simulink model "hdv_hydroelectropowertrain_model"  (R2023b)
settings: Solver=ode1be  StartTime=0.0  StopTime=simulation_length  FixedStep=tsample  MaxStep=tsample
values from neighbouring files (symbols this model uses):
  alpha = 35    [init_model.m]
  Apump = [0 1; 0 0]    [init_model.m]
  available_torque = torque_base+torque_friction_base    [init_model.m]
  Bpump = [0 1]'    [init_model.m]
  btheta_shaft = 2e2    (= 200)    [init_model.m]
  C1 = 10    [init_model.m]
  consumption = [consumption_1, consumption_2, consumption_3, consumption_4,          consumption_5, consumption_6, consumption_7, consumption_8,          consumption_9, consumption_10, consumption_11, consumption_12,          consumption_13, consumption_14, consumption_15, consumption_16          ]    [ic_engine_data.m]
  Cpump = [k 0]    [init_model.m]
  dp_lim = 400    [init_model.m]
  E0 = 3.685    [init_model.m]
  E1 = 0.2156    [init_model.m]
  E2 = 0    [init_model.m]
  E3 = 0    [init_model.m]
  E_1 = -1.031    [init_model.m]
  Elog = -0.05    [init_model.m]
  eta_v_m = 0.98    [init_model.m]
  eta_v_p = 0.97    [init_model.m]
  ki_dp_comp = 1/dp_lim    (= 0.0025)    [init_model.m]
  ki_te_comp = 2/te_lim    [init_model.m]
  kp_ctrl_m = 1    [init_model.m]
  kp_dp_comp = 0.5/dp_lim    (= 0.00125)    [init_model.m]
  kp_te_comp = 1/te_lim    [init_model.m]
  Kpump = acker(Apump,Bpump,poles)    [init_model.m]
  load_blade_enable = 0    [init_model.m]
  Lpump = acker(Apump',Cpump',pole_so)'    [init_model.m]
  M = 125    [init_model.m]
  Ncell = 185    [init_model.m]
  Npump = -1/(Cpump*inv(Apump-Bpump*Kpump)*Bpump)    [init_model.m]
  omega_e_rpm_ref = 1700    [init_model.m]
  omega_l_max_rpm = omega_l_max/(2*pi)*60    (= 50.3075969543)    [init_model.m]
  q1Kalman = tsample^2*1e-2    (= 1e-08)    [init_model.m]
  q2Kalman = tsample^1*1e-1    (= 0.0001)    [init_model.m]
  q3Kalman = 0    [init_model.m]
  Qhr = 400    [init_model.m]
  R0 = 0.015    [init_model.m]
  R1 = 0.015    [init_model.m]
  R_tg = 1.16/2    (= 0.58)    [init_model.m]
  rKalman = 1    [init_model.m]
  rpm_base = [620 700 800 900 1000 1100 1200 1300 1400 1500 1600 1700 1800      1900 2000 2100]    [ic_engine_data.m]
  rpm_consumption = rpm_base    [ic_engine_data.m]
  simulation_length = 245    [init_model.m]
  tau_load = 75e3    (= 75000)    [init_model.m]
  tau_load_max = 1600*41.4    (= 66240)    [init_model.m]
  Tc = tsample    (= 0.001)    [init_model.m]
  torque_base = [max(torque_16_data) max(torque_15_data) max(torque_14_data)      max(torque_13_data) max(torque_12_data) max(torque_11_data)      max(torque_10_data) max(torque_9_data) max(torque_8_data)      max(torque_7_data) max(torque_6_data) max(torque_5_data)      max(torque_4_data) max(torque_3_data) max(torque_2_data)      max(torque_1_data)]    [ic_engine_data.m]
  torque_consumption = torque_reference    [ic_engine_data.m]
  torque_friction_base = -(rpm_base./60*2*pi)*0.25-(rpm_base./60*2*pi).^2*5.2e-4    [ic_engine_data.m]
  tsample = 1e-3    (= 0.001)    [init_model.m]
  v_track1_ref = 8    [init_model.m]
  v_track2_ref = 8    [init_model.m]
  valve_mmorifice_max = 2.75    [init_model.m]
  xv_m_max = 1.2    [init_model.m]
undefined symbols (not defined in the file or in its folder): magnitude
libraries: fl_lib x381, nesl_utility x162, linear_swashplate_ctrl_lib x8, flexshaft_lib x5, bichamber_piston_lib x5, variable_displacement_motor_lib x4, variable_displacement_pump_lib x4, fixed_displacement_pump_lib x4, relief_valve_lib x4, inverse_shuttle_valve_lib x4, hydrostatic_threeway_valve_bichamber_piston_lib x4, hydrostatic_fourway_valve_bichamber_piston_lib x4
(part 4 of 9)

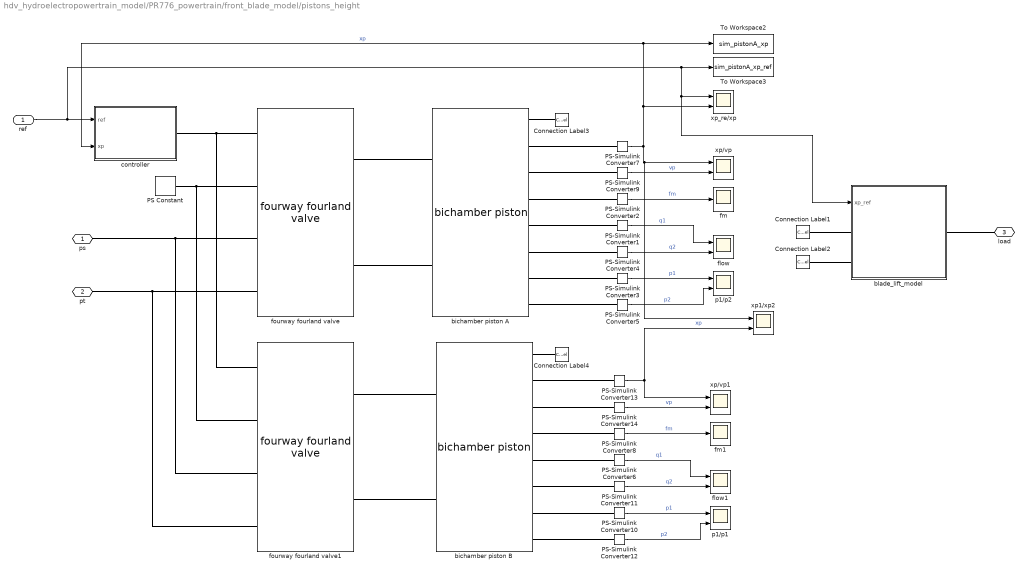
== system hdv_hydroelectropowertrain_model/PR776_powertrain/front_blade_model/pistons_height ==
  ref : Inport
  Connection Label1 : ConnectionLabel  Label=A
  Connection Label2 : ConnectionLabel  Label=B
  Connection Label3 : ConnectionLabel  Label=A
  Connection Label4 : ConnectionLabel  Label=B
  PS Constant : fl_lib/Physical Signals/Sources/PS Constant  constant=0 mm
  PS-Simulink Converter{1..14} (14 alike) : nesl_utility/PS-Simulink Converter  PhysicalDomain=network_engine_domain  SubClassName=ps_output  LeftPortType=input  RightPortType=output  PseudoPeriodic=off  Frequencies=[]  VectorFormat=1-D array  Unit=inherit  AffineConversion=off
  To Workspace2 : ToWorkspace  VariableName=sim_pistonA_xp  SampleTime=Tc
      settings: MaxDataPoints=Nc
  To Workspace3 : ToWorkspace  VariableName=sim_pistonA_xp_ref  SampleTime=Tc
      settings: MaxDataPoints=Nc
  bichamber piston A : bichamber_piston_lib/bichamber piston  A1=8e-3 m^2  A2=8e-3 m^2  Lp=1 m  mp=35 kg  kp=0 N/m  bp=1e3 N/(m/s)  V0=12 l  q1_specify=off  q1_priority=None  q1=0 m^3/s  q1_nominal_specify=off  q1_nominal_unit=m^3/s  q1_nominal_value=1  q2_specify=off  q2_priority=None  q2=0 m^3/s  q2_nominal_specify=off  q2_nominal_unit=m^3/s  q2_nominal_value=1  p1_specify=off  p1_priority=High  p1=0 bar  p1_nominal_specify=off  p1_nominal_unit=bar  p1_nominal_value=1  p2_specify=off  p2_priority=High  p2=125 bar  p2_nominal_specify=off  p2_nominal_unit=bar  p2_nominal_value=1  fp_specify=off  fp_priority=None  fp=0 N  fp_nominal_specify=off  fp_nominal_unit=N  fp_nominal_value=1  vp_specify=off  vp_priority=None  vp=0 m/s  vp_nominal_specify=off  vp_nominal_unit=m/s  vp_nominal_value=1  xp_specify=off  xp_priority=High  xp=0 m  xp_nominal_specify=off  xp_nominal_unit=m  xp_nominal_value=1
      settings: InternalSimscapePortConfiguration="{\"Bottom\":[],\"Left\":[{\"id\":\"H1\",\"label\":\"H1\",\"type\":\"foundation.hydraulic.hydraulic\"},{\"id\":\"H2\",\"label\":\"H2\",\"type\":\"foundation.hydraulic.hydraulic\"}],\"Right\":[{\"id\":\"P\",\"label\":\"P\",\"type\":\"foundation.mechanical.translational.translational\"},{\"id\":\"xp_out\",\"label\":\"xp\",\"type\":\"output\"},{\"id\":\"vp_out\",\"label\":\"vp\",\"type\":\"output\"},{\"id\":\"mforce\",\"label\":\"fm\",\"type\":\"output\"},{\"id\":\"q1_out\",\"label\":\"q1\",\"type\":\"output\"},{\"id\":\"q2_out\",\"label\":\"q2\",\"type\":\"output\"},{\"id\":\"p1_out\",\"label\":\"p1\",\"type\":\"output\"},{\"id\":\"p2_out\",\"label\":\"p2\",\"type\":\"output\"}],\"Top\":[]}"
  bichamber piston B : bichamber_piston_lib/bichamber piston  A1=8e-3 m^2  A2=8e-3 m^2  Lp=1 m  mp=35 kg  kp=0 N/m  bp=1e3 N/(m/s)  V0=12 l  q1_specify=off  q1_priority=None  q1=0 m^3/s  q1_nominal_specify=off  q1_nominal_unit=m^3/s  q1_nominal_value=1  q2_specify=off  q2_priority=None  q2=0 m^3/s  q2_nominal_specify=off  q2_nominal_unit=m^3/s  q2_nominal_value=1  p1_specify=off  p1_priority=High  p1=0 bar  p1_nominal_specify=off  p1_nominal_unit=bar  p1_nominal_value=1  p2_specify=off  p2_priority=High  p2=125 bar  p2_nominal_specify=off  p2_nominal_unit=bar  p2_nominal_value=1  fp_specify=off  fp_priority=None  fp=0 N  fp_nominal_specify=off  fp_nominal_unit=N  fp_nominal_value=1  vp_specify=off  vp_priority=None  vp=0 m/s  vp_nominal_specify=off  vp_nominal_unit=m/s  vp_nominal_value=1  xp_specify=off  xp_priority=High  xp=0 m  xp_nominal_specify=off  xp_nominal_unit=m  xp_nominal_value=1
      settings: InternalSimscapePortConfiguration="{\"Bottom\":[],\"Left\":[{\"id\":\"H1\",\"label\":\"H1\",\"type\":\"foundation.hydraulic.hydraulic\"},{\"id\":\"H2\",\"label\":\"H2\",\"type\":\"foundation.hydraulic.hydraulic\"}],\"Right\":[{\"id\":\"P\",\"label\":\"P\",\"type\":\"foundation.mechanical.translational.translational\"},{\"id\":\"xp_out\",\"label\":\"xp\",\"type\":\"output\"},{\"id\":\"vp_out\",\"label\":\"vp\",\"type\":\"output\"},{\"id\":\"mforce\",\"label\":\"fm\",\"type\":\"output\"},{\"id\":\"q1_out\",\"label\":\"q1\",\"type\":\"output\"},{\"id\":\"q2_out\",\"label\":\"q2\",\"type\":\"output\"},{\"id\":\"p1_out\",\"label\":\"p1\",\"type\":\"output\"},{\"id\":\"p2_out\",\"label\":\"p2\",\"type\":\"output\"}],\"Top\":[]}"
  blade_lift_model : Subsystem
  controller : Subsystem
  flow : Scope  NumInputPorts=2
  flow1 : Scope  NumInputPorts=2
  fm : Scope
  fm1 : Scope
  fourway fourland valve : fourway_fourland_valve_lib/fourway fourland valve  xv_max=valve_mmorifice_max mm  ps_specify=off  ps_priority=None  ps=0 bar  ps_nominal_specify=off  ps_nominal_unit=bar  ps_nominal_value=1  pt_specify=off  pt_priority=None  pt=0 bar  pt_nominal_specify=off  pt_nominal_unit=bar  pt_nominal_value=1  q1_specify=off  q1_priority=None  q1=0 m^3/s  q1_nominal_specify=off  q1_nominal_unit=m^3/s  q1_nominal_value=1  q2_specify=off  q2_priority=None  q2=0 m^3/s  q2_nominal_specify=off  q2_nominal_unit=m^3/s  q2_nominal_value=1  q3_specify=off  q3_priority=None  q3=0 m^3/s  q3_nominal_specify=off  q3_nominal_unit=m^3/s  q3_nominal_value=1  q4_specify=off  q4_priority=None  q4=0 m^3/s  q4_nominal_specify=off  q4_nominal_unit=m^3/s  q4_nominal_value=1  q5_specify=off  q5_priority=None  q5=0 m^3/s  q5_nominal_specify=off  q5_nominal_unit=m^3/s  q5_nominal_value=1  q6_specify=off  q6_priority=None  q6=0 m^3/s  q6_nominal_specify=off  q6_nominal_unit=m^3/s  q6_nominal_value=1  qs_specify=off  qs_priority=None  qs=0 m^3/s  qs_nominal_specify=off  qs_nominal_unit=m^3/s  qs_nominal_value=1  qt_specify=off  qt_priority=None  qt=0 m^3/s  qt_nominal_specify=off  qt_nominal_unit=m^3/s  qt_nominal_value=1  p1_specify=off  p1_priority=High  p1=125 bar  p1_nominal_specify=off  p1_nominal_unit=bar  p1_nominal_value=1  p2_specify=off  p2_priority=High  p2=125 bar  p2_nominal_specify=off  p2_nominal_unit=bar  p2_nominal_value=1
      settings: InternalSimscapePortConfiguration="{\"Bottom\":[],\"Left\":[{\"id\":\"xv\",\"label\":\"xv\",\"type\":\"input\"},{\"id\":\"x0\",\"label\":\"x0\",\"type\":\"input\"},{\"id\":\"S\",\"label\":\"S\",\"type\":\"foundation.hydraulic.hydraulic\"},{\"id\":\"T\",\"label\":\"T\",\"type\":\"foundation.hydraulic.hydraulic\"}],\"Right\":[{\"id\":\"H1\",\"label\":\"H1\",\"type\":\"foundation.hydraulic.hydraulic\"},{\"id\":\"H2\",\"label\":\"H2\",\"type\":\"foundation.hydraulic.hydraulic\"}],\"Top\":[]}"
  fourway fourland valve1 : fourway_fourland_valve_lib/fourway fourland valve  xv_max=valve_mmorifice_max mm  ps_specify=off  ps_priority=None  ps=0 bar  ps_nominal_specify=off  ps_nominal_unit=bar  ps_nominal_value=1  pt_specify=off  pt_priority=None  pt=0 bar  pt_nominal_specify=off  pt_nominal_unit=bar  pt_nominal_value=1  q1_specify=off  q1_priority=None  q1=0 m^3/s  q1_nominal_specify=off  q1_nominal_unit=m^3/s  q1_nominal_value=1  q2_specify=off  q2_priority=None  q2=0 m^3/s  q2_nominal_specify=off  q2_nominal_unit=m^3/s  q2_nominal_value=1  q3_specify=off  q3_priority=None  q3=0 m^3/s  q3_nominal_specify=off  q3_nominal_unit=m^3/s  q3_nominal_value=1  q4_specify=off  q4_priority=None  q4=0 m^3/s  q4_nominal_specify=off  q4_nominal_unit=m^3/s  q4_nominal_value=1  q5_specify=off  q5_priority=None  q5=0 m^3/s  q5_nominal_specify=off  q5_nominal_unit=m^3/s  q5_nominal_value=1  q6_specify=off  q6_priority=None  q6=0 m^3/s  q6_nominal_specify=off  q6_nominal_unit=m^3/s  q6_nominal_value=1  qs_specify=off  qs_priority=None  qs=0 m^3/s  qs_nominal_specify=off  qs_nominal_unit=m^3/s  qs_nominal_value=1  qt_specify=off  qt_priority=None  qt=0 m^3/s  qt_nominal_specify=off  qt_nominal_unit=m^3/s  qt_nominal_value=1  p1_specify=off  p1_priority=High  p1=125 bar  p1_nominal_specify=off  p1_nominal_unit=bar  p1_nominal_value=1  p2_specify=off  p2_priority=High  p2=125 bar  p2_nominal_specify=off  p2_nominal_unit=bar  p2_nominal_value=1
      settings: InternalSimscapePortConfiguration="{\"Bottom\":[],\"Left\":[{\"id\":\"xv\",\"label\":\"xv\",\"type\":\"input\"},{\"id\":\"x0\",\"label\":\"x0\",\"type\":\"input\"},{\"id\":\"S\",\"label\":\"S\",\"type\":\"foundation.hydraulic.hydraulic\"},{\"id\":\"T\",\"label\":\"T\",\"type\":\"foundation.hydraulic.hydraulic\"}],\"Right\":[{\"id\":\"H1\",\"label\":\"H1\",\"type\":\"foundation.hydraulic.hydraulic\"},{\"id\":\"H2\",\"label\":\"H2\",\"type\":\"foundation.hydraulic.hydraulic\"}],\"Top\":[]}"
  p1/p1 : Scope  NumInputPorts=2
  p1/p2 : Scope  NumInputPorts=2
  xp/vp : Scope  NumInputPorts=2
  xp/vp1 : Scope  NumInputPorts=2
  xp1/xp2 : Scope  NumInputPorts=2
  xp_re/xp : Scope  NumInputPorts=2
  ps : PMIOPort  Side=Left
  pt : PMIOPort  Port=2  Side=Left
  load : PMIOPort  Port=3  Side=Right
  wires:
  PS-Simulink Converter3/1 -> p1/p2/1  "p1"
  PS-Simulink Converter7/1 -> controller/2(xp), To Workspace2/1, xp_re/xp/2, xp1/xp2/1, xp/vp/1  "xp"
  PS-Simulink Converter4/1 -> flow/2  "q2"
  PS-Simulink Converter9/1 -> xp/vp/2  "vp"
  PS-Simulink Converter5/1 -> p1/p2/2  "p2"
  PS-Simulink Converter1/1 -> flow/1  "q1"
  PS-Simulink Converter2/1 -> fm/1  "fm"
  PS-Simulink Converter8/1 -> fm1/1  "fm"
  PS-Simulink Converter6/1 -> flow1/1  "q1"
  PS-Simulink Converter12/1 -> p1/p1/2  "p2"
  PS-Simulink Converter14/1 -> xp/vp1/2  "vp"
  PS-Simulink Converter11/1 -> flow1/2  "q2"
  PS-Simulink Converter13/1 -> xp1/xp2/2, xp/vp1/1  "xp"
  PS-Simulink Converter10/1 -> p1/p1/1  "p1"
  ref/1 -> blade_lift_model/1(xp_ref), xp_re/xp/1, To Workspace3/1, controller/1(ref)
  connections:
  bichamber piston A/RConn2 -- PS-Simulink Converter7/LConn1
  bichamber piston A/RConn3 -- PS-Simulink Converter9/LConn1
  bichamber piston A/RConn4 -- PS-Simulink Converter2/LConn1
  bichamber piston A/RConn5 -- PS-Simulink Converter1/LConn1
  bichamber piston A/RConn6 -- PS-Simulink Converter4/LConn1
  bichamber piston A/RConn7 -- PS-Simulink Converter3/LConn1
  bichamber piston A/RConn8 -- PS-Simulink Converter5/LConn1
  bichamber piston A/LConn1 -- fourway fourland valve/RConn1
  bichamber piston A/LConn2 -- fourway fourland valve/RConn2
  ps/RConn1 -- fourway fourland valve1/LConn3 -- fourway fourland valve/LConn3
  pt/RConn1 -- fourway fourland valve1/LConn4 -- fourway fourland valve/LConn4
  controller/RConn1 -- fourway fourland valve1/LConn1 -- fourway fourland valve/LConn1
  PS Constant/RConn1 -- fourway fourland valve/LConn2 -- fourway fourland valve1/LConn2
  bichamber piston B/RConn7 -- PS-Simulink Converter10/LConn1
  bichamber piston B/RConn5 -- PS-Simulink Converter6/LConn1
  bichamber piston B/RConn8 -- PS-Simulink Converter12/LConn1
  bichamber piston B/RConn4 -- PS-Simulink Converter8/LConn1
  bichamber piston B/RConn2 -- PS-Simulink Converter13/LConn1
  bichamber piston B/RConn3 -- PS-Simulink Converter14/LConn1
  bichamber piston B/RConn6 -- PS-Simulink Converter11/LConn1
  fourway fourland valve1/RConn1 -- bichamber piston B/LConn1
  fourway fourland valve1/RConn2 -- bichamber piston B/LConn2
  Connection Label3/LConn1 -- bichamber piston A/RConn1
  Connection Label4/LConn1 -- bichamber piston B/RConn1
  Connection Label1/LConn1 -- blade_lift_model/LConn1
  load/RConn1 -- blade_lift_model/RConn1
  Connection Label2/LConn1 -- blade_lift_model/LConn2

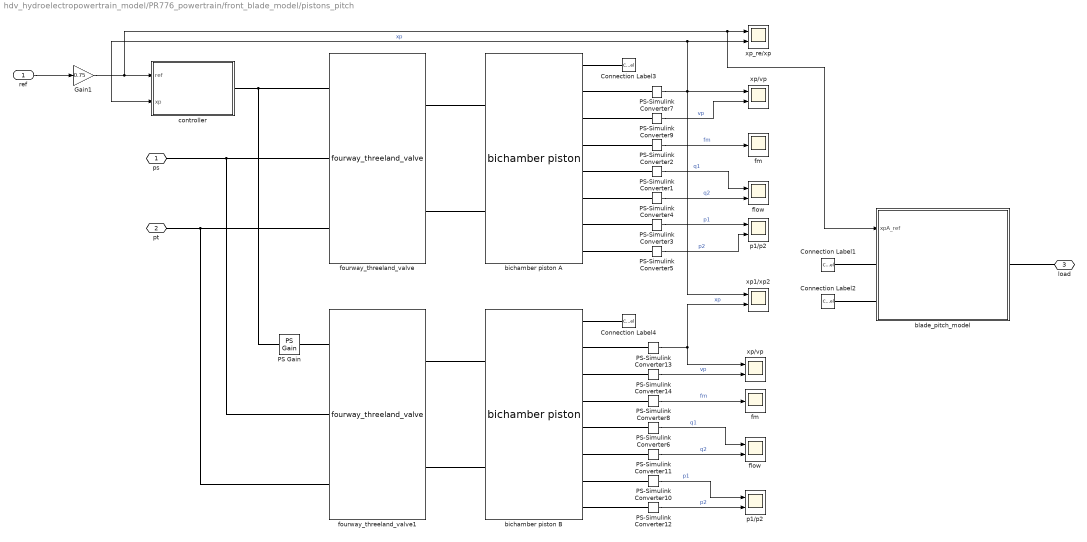
== system hdv_hydroelectropowertrain_model/PR776_powertrain/front_blade_model/pistons_pitch ==
  ref : Inport
  Connection Label1 : ConnectionLabel  Label=A
  Connection Label2 : ConnectionLabel  Label=B
  Connection Label3 : ConnectionLabel  Label=A
  Connection Label4 : ConnectionLabel  Label=B
  Gain1 : Gain  Gain=0.75
  PS Gain : fl_lib/Physical Signals/Functions/PS Gain  gain=-1
  PS-Simulink Converter{1..14} (14 alike) : nesl_utility/PS-Simulink Converter  PhysicalDomain=network_engine_domain  SubClassName=ps_output  LeftPortType=input  RightPortType=output  PseudoPeriodic=off  Frequencies=[]  VectorFormat=1-D array  Unit=inherit  AffineConversion=off
  bichamber piston A : bichamber_piston_lib/bichamber piston  A1=8e-3 m^2  A2=8e-3 m^2  Lp=1.1 m  mp=35 kg  kp=0 N/m  bp=1e3 N/(m/s)  V0=12 l  q1_specify=off  q1_priority=None  q1=0 m^3/s  q1_nominal_specify=off  q1_nominal_unit=m^3/s  q1_nominal_value=1  q2_specify=off  q2_priority=None  q2=0 m^3/s  q2_nominal_specify=off  q2_nominal_unit=m^3/s  q2_nominal_value=1  p1_specify=off  p1_priority=High  p1=0 bar  p1_nominal_specify=off  p1_nominal_unit=bar  p1_nominal_value=1  p2_specify=off  p2_priority=High  p2=0 bar  p2_nominal_specify=off  p2_nominal_unit=bar  p2_nominal_value=1  fp_specify=off  fp_priority=None  fp=0 N  fp_nominal_specify=off  fp_nominal_unit=N  fp_nominal_value=1  vp_specify=off  vp_priority=None  vp=0 m/s  vp_nominal_specify=off  vp_nominal_unit=m/s  vp_nominal_value=1  xp_specify=off  xp_priority=High  xp=0 m  xp_nominal_specify=off  xp_nominal_unit=m  xp_nominal_value=1
      settings: InternalSimscapePortConfiguration="{\"Bottom\":[],\"Left\":[{\"id\":\"H1\",\"label\":\"H1\",\"type\":\"foundation.hydraulic.hydraulic\"},{\"id\":\"H2\",\"label\":\"H2\",\"type\":\"foundation.hydraulic.hydraulic\"}],\"Right\":[{\"id\":\"P\",\"label\":\"P\",\"type\":\"foundation.mechanical.translational.translational\"},{\"id\":\"xp_out\",\"label\":\"xp\",\"type\":\"output\"},{\"id\":\"vp_out\",\"label\":\"vp\",\"type\":\"output\"},{\"id\":\"mforce\",\"label\":\"fm\",\"type\":\"output\"},{\"id\":\"q1_out\",\"label\":\"q1\",\"type\":\"output\"},{\"id\":\"q2_out\",\"label\":\"q2\",\"type\":\"output\"},{\"id\":\"p1_out\",\"label\":\"p1\",\"type\":\"output\"},{\"id\":\"p2_out\",\"label\":\"p2\",\"type\":\"output\"}],\"Top\":[]}"
  bichamber piston B : bichamber_piston_lib/bichamber piston  A1=8e-3 m^2  A2=8e-3 m^2  Lp=1.1 m  mp=35 kg  kp=0 N/m  bp=1e3 N/(m/s)  V0=12 l  q1_specify=off  q1_priority=None  q1=0 m^3/s  q1_nominal_specify=off  q1_nominal_unit=m^3/s  q1_nominal_value=1  q2_specify=off  q2_priority=None  q2=0 m^3/s  q2_nominal_specify=off  q2_nominal_unit=m^3/s  q2_nominal_value=1  p1_specify=off  p1_priority=High  p1=0 bar  p1_nominal_specify=off  p1_nominal_unit=bar  p1_nominal_value=1  p2_specify=off  p2_priority=High  p2=0 bar  p2_nominal_specify=off  p2_nominal_unit=bar  p2_nominal_value=1  fp_specify=off  fp_priority=None  fp=0 N  fp_nominal_specify=off  fp_nominal_unit=N  fp_nominal_value=1  vp_specify=off  vp_priority=None  vp=0 m/s  vp_nominal_specify=off  vp_nominal_unit=m/s  vp_nominal_value=1  xp_specify=off  xp_priority=High  xp=0 m  xp_nominal_specify=off  xp_nominal_unit=m  xp_nominal_value=1
      settings: InternalSimscapePortConfiguration="{\"Bottom\":[],\"Left\":[{\"id\":\"H1\",\"label\":\"H1\",\"type\":\"foundation.hydraulic.hydraulic\"},{\"id\":\"H2\",\"label\":\"H2\",\"type\":\"foundation.hydraulic.hydraulic\"}],\"Right\":[{\"id\":\"P\",\"label\":\"P\",\"type\":\"foundation.mechanical.translational.translational\"},{\"id\":\"xp_out\",\"label\":\"xp\",\"type\":\"output\"},{\"id\":\"vp_out\",\"label\":\"vp\",\"type\":\"output\"},{\"id\":\"mforce\",\"label\":\"fm\",\"type\":\"output\"},{\"id\":\"q1_out\",\"label\":\"q1\",\"type\":\"output\"},{\"id\":\"q2_out\",\"label\":\"q2\",\"type\":\"output\"},{\"id\":\"p1_out\",\"label\":\"p1\",\"type\":\"output\"},{\"id\":\"p2_out\",\"label\":\"p2\",\"type\":\"output\"}],\"Top\":[]}"
  blade_pitch_model : Subsystem
  controller : Subsystem
  flow : Scope  NumInputPorts=2
  "flow " : Scope  NumInputPorts=2
  fm : Scope
  "fm " : Scope
  fourway_threeland_valve : fourway_threeland_valve_lib/fourway_threeland_valve  xv_max=valve_mmorifice_max mm  q1_specify=off  q1_priority=None  q1=0 m^3/s  q1_nominal_specify=off  q1_nominal_unit=m^3/s  q1_nominal_value=1  q2_specify=off  q2_priority=None  q2=0 m^3/s  q2_nominal_specify=off  q2_nominal_unit=m^3/s  q2_nominal_value=1  qin_specify=off  qin_priority=None  qin=0 m^3/s  qin_nominal_specify=off  qin_nominal_unit=m^3/s  qin_nominal_value=1  qout_specify=off  qout_priority=None  qout=0 m^3/s  qout_nominal_specify=off  qout_nominal_unit=m^3/s  qout_nominal_value=1  p1_specify=off  p1_priority=None  p1=0 bar  p1_nominal_specify=off  p1_nominal_unit=bar  p1_nominal_value=1  p2_specify=off  p2_priority=None  p2=0 bar  p2_nominal_specify=off  p2_nominal_unit=bar  p2_nominal_value=1  ps_specify=off  ps_priority=None  ps=0 bar  ps_nominal_specify=off  ps_nominal_unit=bar  ps_nominal_value=1  pt_specify=off  pt_priority=None  pt=0 bar  pt_nominal_specify=off  pt_nominal_unit=bar  pt_nominal_value=1
      settings: InternalSimscapePortConfiguration="{\"Bottom\":[],\"Left\":[{\"id\":\"xv\",\"label\":\"xv\",\"type\":\"input\"},{\"id\":\"S\",\"label\":\"S\",\"type\":\"foundation.hydraulic.hydraulic\"},{\"id\":\"T\",\"label\":\"T\",\"type\":\"foundation.hydraulic.hydraulic\"}],\"Right\":[{\"id\":\"H1\",\"label\":\"H1\",\"type\":\"foundation.hydraulic.hydraulic\"},{\"id\":\"H2\",\"label\":\"H2\",\"type\":\"foundation.hydraulic.hydraulic\"}],\"Top\":[]}"
  fourway_threeland_valve1 : fourway_threeland_valve_lib/fourway_threeland_valve  xv_max=valve_mmorifice_max mm  q1_specify=off  q1_priority=None  q1=0 m^3/s  q1_nominal_specify=off  q1_nominal_unit=m^3/s  q1_nominal_value=1  q2_specify=off  q2_priority=None  q2=0 m^3/s  q2_nominal_specify=off  q2_nominal_unit=m^3/s  q2_nominal_value=1  qin_specify=off  qin_priority=None  qin=0 m^3/s  qin_nominal_specify=off  qin_nominal_unit=m^3/s  qin_nominal_value=1  qout_specify=off  qout_priority=None  qout=0 m^3/s  qout_nominal_specify=off  qout_nominal_unit=m^3/s  qout_nominal_value=1  p1_specify=off  p1_priority=None  p1=0 bar  p1_nominal_specify=off  p1_nominal_unit=bar  p1_nominal_value=1  p2_specify=off  p2_priority=None  p2=0 bar  p2_nominal_specify=off  p2_nominal_unit=bar  p2_nominal_value=1  ps_specify=off  ps_priority=None  ps=0 bar  ps_nominal_specify=off  ps_nominal_unit=bar  ps_nominal_value=1  pt_specify=off  pt_priority=None  pt=0 bar  pt_nominal_specify=off  pt_nominal_unit=bar  pt_nominal_value=1
      settings: InternalSimscapePortConfiguration="{\"Bottom\":[],\"Left\":[{\"id\":\"xv\",\"label\":\"xv\",\"type\":\"input\"},{\"id\":\"S\",\"label\":\"S\",\"type\":\"foundation.hydraulic.hydraulic\"},{\"id\":\"T\",\"label\":\"T\",\"type\":\"foundation.hydraulic.hydraulic\"}],\"Right\":[{\"id\":\"H1\",\"label\":\"H1\",\"type\":\"foundation.hydraulic.hydraulic\"},{\"id\":\"H2\",\"label\":\"H2\",\"type\":\"foundation.hydraulic.hydraulic\"}],\"Top\":[]}"
  p1/p2 : Scope  NumInputPorts=2
  "p1/p2 " : Scope  NumInputPorts=2
  xp/vp : Scope  NumInputPorts=2
  "xp/vp " : Scope  NumInputPorts=2
  xp1/xp2 : Scope  NumInputPorts=2
  xp_re/xp : Scope  NumInputPorts=2
  ps : PMIOPort  Side=Left
  pt : PMIOPort  Port=2  Side=Left
  load : PMIOPort  Port=3  Side=Right
  wires:
  PS-Simulink Converter10/1 -> "p1/p2 "/1  "p1"
  PS-Simulink Converter13/1 -> xp1/xp2/2, "xp/vp "/1  "xp"
  PS-Simulink Converter11/1 -> "flow "/2  "q2"
  PS-Simulink Converter14/1 -> "xp/vp "/2  "vp"
  PS-Simulink Converter12/1 -> "p1/p2 "/2  "p2"
  PS-Simulink Converter6/1 -> "flow "/1  "q1"
  PS-Simulink Converter8/1 -> "fm "/1  "fm"
  PS-Simulink Converter2/1 -> fm/1  "fm"
  PS-Simulink Converter1/1 -> flow/1  "q1"
  PS-Simulink Converter5/1 -> p1/p2/2  "p2"
  PS-Simulink Converter9/1 -> xp/vp/2  "vp"
  PS-Simulink Converter4/1 -> flow/2  "q2"
  PS-Simulink Converter7/1 -> xp1/xp2/1, xp/vp/1, controller/2(xp), xp_re/xp/2  "xp"
  PS-Simulink Converter3/1 -> p1/p2/1  "p1"
  ref/1 -> Gain1/1
  Gain1/1 -> controller/1(ref), blade_pitch_model/1(xpA_ref), xp_re/xp/1
  connections:
  bichamber piston B/RConn6 -- PS-Simulink Converter11/LConn1
  bichamber piston B/RConn3 -- PS-Simulink Converter14/LConn1
  bichamber piston B/RConn2 -- PS-Simulink Converter13/LConn1
  bichamber piston B/RConn4 -- PS-Simulink Converter8/LConn1
  bichamber piston B/RConn8 -- PS-Simulink Converter12/LConn1
  bichamber piston B/RConn5 -- PS-Simulink Converter6/LConn1
  bichamber piston B/RConn7 -- PS-Simulink Converter10/LConn1
  fourway_threeland_valve/LConn1 -- PS Gain/LConn1 -- controller/RConn1
  pt/RConn1 -- fourway_threeland_valve/LConn3 -- fourway_threeland_valve1/LConn3
  ps/RConn1 -- fourway_threeland_valve/LConn2 -- fourway_threeland_valve1/LConn2
  bichamber piston A/RConn8 -- PS-Simulink Converter5/LConn1
  bichamber piston A/RConn7 -- PS-Simulink Converter3/LConn1
  bichamber piston A/RConn6 -- PS-Simulink Converter4/LConn1
  bichamber piston A/RConn5 -- PS-Simulink Converter1/LConn1
  bichamber piston A/RConn4 -- PS-Simulink Converter2/LConn1
  bichamber piston A/RConn2 -- PS-Simulink Converter7/LConn1
  bichamber piston A/LConn1 -- fourway_threeland_valve/RConn1
  bichamber piston A/LConn2 -- fourway_threeland_valve/RConn2
  PS Gain/RConn1 -- fourway_threeland_valve1/LConn1
  bichamber piston A/RConn3 -- PS-Simulink Converter9/LConn1
  fourway_threeland_valve1/RConn1 -- bichamber piston B/LConn1
  fourway_threeland_valve1/RConn2 -- bichamber piston B/LConn2
  Connection Label3/LConn1 -- bichamber piston A/RConn1
  bichamber piston B/RConn1 -- Connection Label4/LConn1
  Connection Label1/LConn1 -- blade_pitch_model/LConn1
  Connection Label2/LConn1 -- blade_pitch_model/LConn2
  blade_pitch_model/RConn1 -- load/RConn1

== system hdv_hydroelectropowertrain_model/PR776_powertrain/front_blade_model/pitch_load ==
  Simulink-PS Converter1 : nesl_utility/Simulink-PS Converter  PhysicalDomain=network_engine_domain  SubClassName=ps_input  LeftPortType=input  RightPortType=output  PseudoPeriodic=off  Frequencies=[]  NoiseDistribution=none  NoiseParameters=[]  Unit=N  AffineConversion=on  FilteringAndDerivatives=provide  SimscapeFilterOrder=1  InputFilterTimeConstant=0.001  UdotUserProvided=0
  "pitch_load  " : Subsystem
  load : PMIOPort  Side=Right
  wires:
  "pitch_load  "/1(Out1) -> Simulink-PS Converter1/1  "pitch_load"
  connections:
  load/RConn1 -- Simulink-PS Converter1/RConn1

== system hdv_hydroelectropowertrain_model/PR776_powertrain/front_blade_model/tilt_load ==
  Simulink-PS Converter1 : nesl_utility/Simulink-PS Converter  PhysicalDomain=network_engine_domain  SubClassName=ps_input  LeftPortType=input  RightPortType=output  PseudoPeriodic=off  Frequencies=[]  NoiseDistribution=none  NoiseParameters=[]  Unit=N  AffineConversion=on  FilteringAndDerivatives=provide  SimscapeFilterOrder=1  InputFilterTimeConstant=0.001  UdotUserProvided=0
  "tilt_load  " : Subsystem
  load : PMIOPort  Side=Right
  wires:
  "tilt_load  "/1(Out1) -> Simulink-PS Converter1/1  "tilt_load"
  connections:
  load/RConn1 -- Simulink-PS Converter1/RConn1

== system hdv_hydroelectropowertrain_model/PR776_powertrain/front_blade_model/vertical_load ==
  Blade_load : fl_lib/Mechanical/Mechanical Sources/Ideal Force Source
  Constant : Constant  Value=31878
  Mechanical Translational Reference : fl_lib/Mechanical/Translational Elements/Mechanical Translational Reference
  Simulink-PS Converter1 : nesl_utility/Simulink-PS Converter  PhysicalDomain=network_engine_domain  SubClassName=ps_input  LeftPortType=input  RightPortType=output  PseudoPeriodic=off  Frequencies=[]  NoiseDistribution=none  NoiseParameters=[]  Unit=N  AffineConversion=on  FilteringAndDerivatives=provide  SimscapeFilterOrder=1  InputFilterTimeConstant=0.001  UdotUserProvided=0
  To Workspace6 : ToWorkspace  VariableName=sim_load  SampleTime=Tc
      settings: MaxDataPoints=Nc
  load : Scope
  load_disturbance : Subsystem
  vertical_load : PMIOPort  Side=Left
  wires:
  load_disturbance/1(Out1) -> load/1, To Workspace6/1  "load_force"
  Constant/1 -> Simulink-PS Converter1/1
  connections:
  Mechanical Translational Reference/LConn1 -- Blade_load/RConn2
  Simulink-PS Converter1/RConn1 -- Blade_load/RConn1
  vertical_load/RConn1 -- Blade_load/LConn1

== system hdv_hydroelectropowertrain_model/Vehicle Control System/Engine Anti-Stall/Engine Overload Control ==
  x : Inport
  xref : Inport  Port=2
  1/Ti : Gain  Gain=kp  SaturateOnIntegerOverflow=on  OutDataTypeStr=Inherit: Same as input  ParamDataTypeStr=Inherit: Same as input
  Saturation : Saturate  UpperLimit=sat_pos  LowerLimit=sat_neg
  Sum1 : Sum  Inputs=+++  SaturateOnIntegerOverflow=on
  Sum2 : Sum  Inputs=-+  SaturateOnIntegerOverflow=on
  Sum3 : Sum  Inputs=-+  SaturateOnIntegerOverflow=on
  Unit Delay4 : UnitDelay  SampleTime=tsample  HasFrameUpgradeWarning=on
  kp : Gain  Gain=ki*ts  SaturateOnIntegerOverflow=on  OutDataTypeStr=Inherit: Same as input  ParamDataTypeStr=Inherit: Same as input
  u : Outport
  wires:
  Saturation/1 -> Sum3/2, u/1
  Unit Delay4/1 -> Sum1/3
  Sum1/1 -> Saturation/1
  x/1 -> Sum2/1
  Sum3/1 -> Unit Delay4/1
  1/Ti/1 -> Sum3/1, Sum1/1
  Sum2/1 -> 1/Ti/1, kp/1
  kp/1 -> Sum1/2
  xref/1 -> Sum2/2

== system hdv_hydroelectropowertrain_model/Vehicle Control System/Over Pressure Compensation/Pressure Compensation Control A ==
  x : Inport
  xref : Inport  Port=2
  1/Ti : Gain  Gain=kp  SaturateOnIntegerOverflow=on  OutDataTypeStr=Inherit: Same as input  ParamDataTypeStr=Inherit: Same as input
  Saturation : Saturate  UpperLimit=sat_pos  LowerLimit=sat_neg
  Sum1 : Sum  Inputs=+++  SaturateOnIntegerOverflow=on
  Sum2 : Sum  Inputs=-+  SaturateOnIntegerOverflow=on
  Sum3 : Sum  Inputs=-+  SaturateOnIntegerOverflow=on
  Unit Delay4 : UnitDelay  SampleTime=tsample  HasFrameUpgradeWarning=on
  kp : Gain  Gain=ki*ts  SaturateOnIntegerOverflow=on  OutDataTypeStr=Inherit: Same as input  ParamDataTypeStr=Inherit: Same as input
  u : Outport
  wires:
  xref/1 -> Sum2/2
  kp/1 -> Sum1/2
  1/Ti/1 -> Sum1/1, Sum3/1
  Sum3/1 -> Unit Delay4/1
  x/1 -> Sum2/1
  Sum1/1 -> Saturation/1
  Unit Delay4/1 -> Sum1/3
  Saturation/1 -> u/1, Sum3/2
  Sum2/1 -> 1/Ti/1, kp/1

== system hdv_hydroelectropowertrain_model/Vehicle Control System/Over Pressure Compensation/Pressure Compensation Control B ==
  x : Inport
  xref : Inport  Port=2
  1/Ti : Gain  Gain=kp  SaturateOnIntegerOverflow=on  OutDataTypeStr=Inherit: Same as input  ParamDataTypeStr=Inherit: Same as input
  Saturation : Saturate  UpperLimit=sat_pos  LowerLimit=sat_neg
  Sum1 : Sum  Inputs=+++  SaturateOnIntegerOverflow=on
  Sum2 : Sum  Inputs=-+  SaturateOnIntegerOverflow=on
  Sum3 : Sum  Inputs=-+  SaturateOnIntegerOverflow=on
  Unit Delay4 : UnitDelay  SampleTime=tsample  HasFrameUpgradeWarning=on
  kp : Gain  Gain=ki*ts  SaturateOnIntegerOverflow=on  OutDataTypeStr=Inherit: Same as input  ParamDataTypeStr=Inherit: Same as input
  u : Outport
  wires:
  Saturation/1 -> Sum3/2, u/1
  Unit Delay4/1 -> Sum1/3
  Sum1/1 -> Saturation/1
  x/1 -> Sum2/1
  Sum3/1 -> Unit Delay4/1
  1/Ti/1 -> Sum3/1, Sum1/1
  Sum2/1 -> 1/Ti/1, kp/1
  kp/1 -> Sum1/2
  xref/1 -> Sum2/2

== system hdv_hydroelectropowertrain_model/Vehicle Control System/Over Pressure Compensation/direction1 ==
  In1 : Inport
  Product : Product
  Out1 : Outport
  wires:
  In1/1 -> Product/1
  Product/1 -> Out1/1
  [direction_RT] -> Product/2

== system hdv_hydroelectropowertrain_model/Vehicle Control System/Over Pressure Compensation/direction2 ==
  In1 : Inport
  Product : Product
  Out1 : Outport
  wires:
  Product/1 -> Out1/1
  In1/1 -> Product/1
  [direction_LT] -> Product/2

== system hdv_hydroelectropowertrain_model/Vehicle Control System/lineA_compensations/direction_RT ==
  In1 : Inport
  Product : Product
  ETComp : Outport
  wires:
  Product/1 -> ETComp/1
  In1/1 -> Product/1
  [direction_RT] -> Product/2

== system hdv_hydroelectropowertrain_model/Vehicle Control System/lineB_compensations /direction_LT ==
  In1 : Inport
  Product : Product
  ETComp : Outport
  wires:
  Product/1 -> ETComp/1
  In1/1 -> Product/1
  [direction_LT] -> Product/2

== system hdv_hydroelectropowertrain_model/Vehicle Control System/synch_overspeed_management/Maximum Speed Control ==
  x : Inport
  xref : Inport  Port=2
  1/Ti : Gain  Gain=kp  SaturateOnIntegerOverflow=on  OutDataTypeStr=Inherit: Same as input  ParamDataTypeStr=Inherit: Same as input
  Saturation : Saturate  UpperLimit=sat_pos  LowerLimit=sat_neg
  Sum1 : Sum  Inputs=+++  SaturateOnIntegerOverflow=on
  Sum2 : Sum  Inputs=-+  SaturateOnIntegerOverflow=on
  Sum3 : Sum  Inputs=-+  SaturateOnIntegerOverflow=on
  Unit Delay4 : UnitDelay  SampleTime=ts  HasFrameUpgradeWarning=on
  direction_lineA : Subsystem
  kp : Gain  Gain=ki*tsample  SaturateOnIntegerOverflow=on  OutDataTypeStr=Inherit: Same as input  ParamDataTypeStr=Inherit: Same as input
  u : Outport
  wires:
  xref/1 -> Sum2/2
  kp/1 -> Sum1/2
  1/Ti/1 -> Sum1/1, Sum3/1
  Sum3/1 -> Unit Delay4/1
  x/1 -> Sum2/1
  Sum1/1 -> Saturation/1
  Unit Delay4/1 -> Sum1/3
  Saturation/1 -> direction_lineA/1(In1), Sum3/2
  Sum2/1 -> kp/1, 1/Ti/1
  direction_lineA/1(u) -> u/1

== system hdv_hydroelectropowertrain_model/Vehicle Control System/synch_overspeed_management/Steering Reference Control ==
  x : Inport
  xref : Inport  Port=2
  1/Ti : Gain  Gain=kp  SaturateOnIntegerOverflow=on  OutDataTypeStr=Inherit: Same as input  ParamDataTypeStr=Inherit: Same as input
  Saturation : Saturate  UpperLimit=sat_pos  LowerLimit=sat_neg
  Sum1 : Sum  Inputs=+++  SaturateOnIntegerOverflow=on
  Sum2 : Sum  Inputs=-+  SaturateOnIntegerOverflow=on
  Sum3 : Sum  Inputs=-+  SaturateOnIntegerOverflow=on
  Unit Delay4 : UnitDelay  SampleTime=tsample  HasFrameUpgradeWarning=on
  kp : Gain  Gain=ki*ts  SaturateOnIntegerOverflow=on  OutDataTypeStr=Inherit: Same as input  ParamDataTypeStr=Inherit: Same as input
  u : Outport
  wires:
  Saturation/1 -> Sum3/2, u/1
  Unit Delay4/1 -> Sum1/3
  Sum1/1 -> Saturation/1
  x/1 -> Sum2/1
  Sum3/1 -> Unit Delay4/1
  1/Ti/1 -> Sum3/1, Sum1/1
  Sum2/1 -> 1/Ti/1, kp/1
  kp/1 -> Sum1/2
  xref/1 -> Sum2/2

== system hdv_hydroelectropowertrain_model/PR776_powertrain/Hydrostatic_powertrain/driveine_LD1/pressure_charge_system_LD ==
  Hydraulic Flow Rate Sensor : fl_lib/Hydraulic/Hydraulic Sensors/Hydraulic Flow Rate Sensor
  Hydraulic Flow Rate Sensor1 : fl_lib/Hydraulic/Hydraulic Sensors/Hydraulic Flow Rate Sensor
  Hydraulic Pressure Sensor{1..4} (4 alike) : fl_lib/Hydraulic/Hydraulic Sensors/Hydraulic Pressure Sensor
  Hydraulic Reference1 : fl_lib/Hydraulic/Hydraulic Elements/Hydraulic Reference
  Hydraulic Reference2 : fl_lib/Hydraulic/Hydraulic Elements/Hydraulic Reference
  Hydraulic Reference3 : fl_lib/Hydraulic/Hydraulic Elements/Hydraulic Reference
  Mux : Mux  Inputs=2
  PS-Simulink Converter : nesl_utility/PS-Simulink Converter  PhysicalDomain=network_engine_domain  SubClassName=ps_output  LeftPortType=input  RightPortType=output  PseudoPeriodic=off  Frequencies=[]  VectorFormat=1-D array  Unit=l/min  AffineConversion=on
  PS-Simulink Converter{1..3,5} (4 alike) : nesl_utility/PS-Simulink Converter  PhysicalDomain=network_engine_domain  SubClassName=ps_output  LeftPortType=input  RightPortType=output  PseudoPeriodic=off  Frequencies=[]  VectorFormat=1-D array  Unit=bar  AffineConversion=on
  PS-Simulink Converter4 : nesl_utility/PS-Simulink Converter  PhysicalDomain=network_engine_domain  SubClassName=ps_output  LeftPortType=input  RightPortType=output  PseudoPeriodic=off  Frequencies=[]  VectorFormat=1-D array  Unit=l/min  AffineConversion=on
  Scope1 : Scope  NumInputPorts=2
  Scope2 : Scope  NumInputPorts=2
  Scope3 : Scope  NumInputPorts=2
  Subsystem : Subsystem
  hydro_check_valve1 : Subsystem
      settings: PortSchema="{\"entries\":[{\"content\":{\"sides\":[{\"content\":{\"connectorIds\":[]},\"type\":\"ConnectorPlacement.EquallySpacedRectSide\",\"uuid\":\"a69fbb91-2279-4dfd-af6f-16497d5f1538\"},{\"content\":{\"connectorIds\":[],\"side\":\"RIGHT\"},\"type\":\"ConnectorPlacement.EquallySpacedRectSide\",\"uuid\":\"52e95d44-b7af-4ccc-8556-a2abd2e724e0\"},{\"content\":{\"connectorIds\":[\"LConn1\"],\"side\":\"TOP\"},\"type\":\"ConnectorPlacement.EquallySpacedRectSide\",\"uuid\":\"2d8c071e-4cd0-4b83-8d45-c175cb858754\"},{\"content\":{\"connectorIds\":[\"RConn1\"],\"side\":\"BOTTOM\"},\"type\":\"ConnectorPlacement.EquallySpacedRectSide\",\"uuid\":\"1baec9dc-757c-4f21-904a-6fc08de72ce1\"}]},\"type\":\"ConnectorPlacement.EquallySpacedConnector\",\"uuid\":\"76990e53-6cb0-4bfe-8c9e-427c41b785f2\"}],\"packageUris\":[\"http://schema.mathworks.com/mf0/Connector/19700101\"],\"version\":\"1.0\"}"
  hydro_check_valve2 : Subsystem
      settings: PortSchema="{\"entries\":[{\"content\":{\"sides\":[{\"content\":{\"connectorIds\":[]},\"type\":\"ConnectorPlacement.EquallySpacedRectSide\",\"uuid\":\"a69fbb91-2279-4dfd-af6f-16497d5f1538\"},{\"content\":{\"connectorIds\":[],\"side\":\"RIGHT\"},\"type\":\"ConnectorPlacement.EquallySpacedRectSide\",\"uuid\":\"52e95d44-b7af-4ccc-8556-a2abd2e724e0\"},{\"content\":{\"connectorIds\":[\"LConn1\"],\"side\":\"TOP\"},\"type\":\"ConnectorPlacement.EquallySpacedRectSide\",\"uuid\":\"2d8c071e-4cd0-4b83-8d45-c175cb858754\"},{\"content\":{\"connectorIds\":[\"RConn1\"],\"side\":\"BOTTOM\"},\"type\":\"ConnectorPlacement.EquallySpacedRectSide\",\"uuid\":\"1baec9dc-757c-4f21-904a-6fc08de72ce1\"}]},\"type\":\"ConnectorPlacement.EquallySpacedConnector\",\"uuid\":\"76990e53-6cb0-4bfe-8c9e-427c41b785f2\"}],\"packageUris\":[\"http://schema.mathworks.com/mf0/Connector/19700101\"],\"version\":\"1.0\"}"
  inverse shuttle valve : inverse_shuttle_valve_lib/inverse shuttle valve  pnom=32 bar  dp_crack=0 bar  dp_reg=0 bar  x_rv_max=2 mm  a0=(2*pi*10)^2 1/s^2  a1=2*2*pi*10 1/s  leak=5e-12 m^3/s/Pa  qA_specify=off  qA_priority=None  qA=0 m^3/s  qA_nominal_specify=off  qA_nominal_unit=m^3/s  qA_nominal_value=1  qB_specify=off  qB_priority=None  qB=0 m^3/s  qB_nominal_specify=off  qB_nominal_unit=m^3/s  qB_nominal_value=1  qP_specify=off  qP_priority=None  qP=0 m^3/s  qP_nominal_specify=off  qP_nominal_unit=m^3/s  qP_nominal_value=1  dp_specify=off  dp_priority=None  dp=0 Pa  dp_nominal_specify=off  dp_nominal_unit=Pa  dp_nominal_value=1  dpAP_specify=off  dpAP_priority=None  dpAP=0 Pa  dpAP_nominal_specify=off  dpAP_nominal_unit=Pa  dpAP_nominal_value=1  dpBP_specify=off  dpBP_priority=None  dpBP=0 Pa  dpBP_nominal_specify=off  dpBP_nominal_unit=Pa  dpBP_nominal_value=1  x_rv_AP_specify=off  x_rv_AP_priority=None  x_rv_AP=0 m  x_rv_AP_nominal_specify=off  x_rv_AP_nominal_unit=m  x_rv_AP_nominal_value=1  x_rv_BP_specify=off  x_rv_BP_priority=None  x_rv_BP=0 m  x_rv_BP_nominal_specify=off  x_rv_BP_nominal_unit=m  x_rv_BP_nominal_value=1  x_rv_AP_flt_specify=off  x_rv_AP_flt_priority=None  x_rv_AP_flt=0 m  x_rv_AP_flt_nominal_specify=off  x_rv_AP_flt_nominal_unit=m  x_rv_AP_flt_nominal_value=1  x_rv_BP_flt_specify=off  x_rv_BP_flt_priority=None  x_rv_BP_flt=0 m  x_rv_BP_flt_nominal_specify=off  x_rv_BP_flt_nominal_unit=m  x_rv_BP_flt_nominal_value=1
      settings: InternalSimscapePortConfiguration="{\"Bottom\":[],\"Left\":[{\"id\":\"cA\",\"label\":\"cA\",\"type\":\"foundation.hydraulic.hydraulic\"},{\"id\":\"cB\",\"label\":\"cB\",\"type\":\"foundation.hydraulic.hydraulic\"}],\"Right\":[{\"id\":\"cP\",\"label\":\"cP\",\"type\":\"foundation.hydraulic.hydraulic\"}],\"Top\":[]}"
  A : PMIOPort  Side=Left
  B : PMIOPort  Port=2  Side=Right
  D : PMIOPort  Port=3  Side=Right
  wires:
  PS-Simulink Converter5/1 -> Scope3/2  "dp"
  PS-Simulink Converter4/1 -> Scope3/1  "qT_ishuttle"
  PS-Simulink Converter3/1 -> Scope2/2  "pCharge"
  PS-Simulink Converter/1 -> Scope1/2, Scope2/1  "qcharge"
  Mux/1 -> Scope1/1
  PS-Simulink Converter1/1 -> Mux/1  "pB"
  PS-Simulink Converter2/1 -> Mux/2  "pA"
  connections:
  PS-Simulink Converter5/LConn1 -- Hydraulic Pressure Sensor4/RConn2
  Hydraulic Flow Rate Sensor1/RConn1 -- PS-Simulink Converter4/LConn1
  Hydraulic Flow Rate Sensor1/RConn2 -- Hydraulic Reference3/LConn1
  Hydraulic Reference2/LConn1 -- Hydraulic Pressure Sensor3/RConn1
  Hydraulic Pressure Sensor3/RConn2 -- PS-Simulink Converter3/LConn1
  Subsystem/LConn1 -- D/RConn1
  Hydraulic Flow Rate Sensor/LConn1 -- Subsystem/RConn1 -- Hydraulic Pressure Sensor3/LConn1
  Hydraulic Flow Rate Sensor/RConn1 -- PS-Simulink Converter/LConn1
  Hydraulic Pressure Sensor2/RConn2 -- PS-Simulink Converter2/LConn1
  Hydraulic Pressure Sensor1/RConn2 -- PS-Simulink Converter1/LConn1
  Hydraulic Pressure Sensor1/RConn1 -- Hydraulic Reference1/LConn1 -- Hydraulic Pressure Sensor2/RConn1
  Hydraulic Pressure Sensor4/RConn1 -- Hydraulic Pressure Sensor1/LConn1 -- B/RConn1 -- inverse shuttle valve/LConn2 -- hydro_check_valve2/RConn1
  Hydraulic Pressure Sensor4/LConn1 -- Hydraulic Pressure Sensor2/LConn1 -- A/RConn1 -- inverse shuttle valve/LConn1 -- hydro_check_valve1/RConn1
  hydro_check_valve1/LConn1 -- Hydraulic Flow Rate Sensor/RConn2 -- hydro_check_valve2/LConn1
  inverse shuttle valve/RConn1 -- Hydraulic Flow Rate Sensor1/LConn1

== system hdv_hydroelectropowertrain_model/PR776_powertrain/Hydrostatic_powertrain/driveine_LD1/vd_ctrl_motor_LD ==
  vd_ref : Inport
  Linear swashplate ctrl2 : linear_swashplate_ctrl_lib/Linear swashplate ctrl  Commented=on  a12=1 1/s  b2=1 1/m/s  k1=100 m  k2=20.5 m  N=5 m  kv=20  xv_specify=off  xv_priority=None  xv=0 m  xv_nominal_specify=off  xv_nominal_unit=m  xv_nominal_value=1  D1_specify=off  D1_priority=None  D1=0  D1_nominal_specify=off  D1_nominal_unit=1  D1_nominal_value=1  D2_specify=off  D2_priority=None  D2=0  D2_nominal_specify=off  D2_nominal_unit=1  D2_nominal_value=1
      settings: InternalSimscapePortConfiguration="{\"Bottom\":[],\"Left\":[{\"id\":\"D_ref\",\"label\":\"Dref\",\"type\":\"input\"}],\"Right\":[{\"id\":\"Dout\",\"label\":\"Dout\",\"type\":\"output\"}],\"Top\":[]}"
  PS-Simulink Converter : nesl_utility/PS-Simulink Converter  PhysicalDomain=network_engine_domain  SubClassName=ps_output  LeftPortType=input  RightPortType=output  PseudoPeriodic=off  Frequencies=[]  VectorFormat=1-D array  Unit=inherit  AffineConversion=off
  Scope : Scope  NumInputPorts=2
  Simulink-PS Converter3 : nesl_utility/Simulink-PS Converter  Commented=on  PhysicalDomain=network_engine_domain  SubClassName=ps_input  LeftPortType=input  RightPortType=output  PseudoPeriodic=off  Frequencies=[]  NoiseDistribution=none  NoiseParameters=[]  Unit=1  AffineConversion=off  FilteringAndDerivatives=provide  SimscapeFilterOrder=1  InputFilterTimeConstant=0.001  UdotUserProvided=0
  hose3 : Subsystem
  servo motor LD : Subsystem
  vd : PMIOPort  Side=Right
  pS : PMIOPort  Port=2  Side=Left
  pT : PMIOPort  Port=3  Side=Left
  wires:
  PS-Simulink Converter/1 -> Scope/2
  vd_ref/1 -> servo motor LD/1(displacement reference pu), Scope/1, Simulink-PS Converter3/1
  connections:
  Simulink-PS Converter3/RConn1 -- Linear swashplate ctrl2/LConn1
  pS/RConn1 -- hose3/LConn1
  pT/RConn1 -- hose3/LConn2
  hose3/RConn1 -- servo motor LD/LConn1
  hose3/RConn2 -- servo motor LD/LConn2
  servo motor LD/RConn1 -- PS-Simulink Converter/LConn1 -- vd/RConn1

== system hdv_hydroelectropowertrain_model/PR776_powertrain/Hydrostatic_powertrain/driveine_LD1/vd_ctrl_pump_LD ==
  vd_ref : Inport
  Linear swashplate ctrl2 : linear_swashplate_ctrl_lib/Linear swashplate ctrl  Commented=on  a12=1 1/s  b2=1 1/m/s  k1=100 m  k2=20.5 m  N=5 m  kv=20  xv_specify=off  xv_priority=None  xv=0 m  xv_nominal_specify=off  xv_nominal_unit=m  xv_nominal_value=1  D1_specify=off  D1_priority=None  D1=0  D1_nominal_specify=off  D1_nominal_unit=1  D1_nominal_value=1  D2_specify=off  D2_priority=None  D2=0  D2_nominal_specify=off  D2_nominal_unit=1  D2_nominal_value=1
      settings: InternalSimscapePortConfiguration="{\"Bottom\":[],\"Left\":[{\"id\":\"D_ref\",\"label\":\"Dref\",\"type\":\"input\"}],\"Right\":[{\"id\":\"Dout\",\"label\":\"Dout\",\"type\":\"output\"}],\"Top\":[]}"
  Simulink-PS Converter3 : nesl_utility/Simulink-PS Converter  Commented=on  PhysicalDomain=network_engine_domain  SubClassName=ps_input  LeftPortType=input  RightPortType=output  PseudoPeriodic=off  Frequencies=[]  NoiseDistribution=none  NoiseParameters=[]  Unit=1  AffineConversion=off  FilteringAndDerivatives=provide  SimscapeFilterOrder=1  InputFilterTimeConstant=0.001  UdotUserProvided=0
  hose3 : Subsystem
  servo pump RD : Subsystem
  vd : PMIOPort  Side=Right
  pS : PMIOPort  Port=2  Side=Left
  pT : PMIOPort  Port=3  Side=Left
  wires:
  vd_ref/1 -> Simulink-PS Converter3/1, servo pump RD/1(displacement reference pu)
  connections:
  pT/RConn1 -- hose3/LConn2
  pS/RConn1 -- hose3/LConn1
  servo pump RD/LConn1 -- hose3/RConn1
  servo pump RD/LConn2 -- hose3/RConn2
  Simulink-PS Converter3/RConn1 -- Linear swashplate ctrl2/LConn1
  servo pump RD/RConn1 -- vd/RConn1
